simulink model "VELOCIDAD_COMP"  (R2015a)
settings: Solver=ode3  SolverMode=SingleTasking  StartTime=0.0  StopTime=inf  RelTol=1e-3
InitFcn:
  | % Periodo de muestreo control
  | % Periodo de muestreo control logico
  | tc=ts;
  | % Periodo de muestreo registro
  | tr=5e-3;
  | % Radio de la rueda (m)
  | R=86.1e-3/2;
  | % Distancia entre ruedas (m)
  | W=0.160;
  | % Constante de tiempo de filtrado
  | Tf_vel=200e-3; % Velocidad
values from neighbouring files (symbols this model uses):
  Cd = K*(1+1/(Ti*sd)+(Td*sd)/(1+Td*sd/N))    [ControlP.m]    (also in dead_2015.m = minreal(Fd/Pd/(1-Fd)); p4_3_diseño_directo.m = minreal(F/(Pd-F*Pd)))
  Crd = Cd    [ControlP.m]    (also in dead_2015.m; p4_3_diseño_directo.m)
  ts = 0.5    [ControlP.m]    (also in ControlPID_RF.m = 0.005; dead_2015.m = 0.055)
undefined symbols (not defined in the file or in its folder): Normalized
libraries: legonxtlib x10, simulink x6
settings Model: SimulationMode=external  CovSFcnEnable=off  ExtModeTrigDuration=2  Creator=mogimenez  LastModifiedBy=201809800
settings DataIOCC: SignalLoggingSaveFormat=ModelDataLogs
settings OptimizationCC: ExpressionDepthLimit=2147483647  OptimizeModelRefInitCode=on  LifeSpan=1
settings DebuggingCC: UnderspecifiedInitializationDetection=Classic  MergeDetectMultiDrivingBlocksExec=none  FcnCallInpInsideContextMsg=EnableAllAsWarning  StateNameClashWarn=warning
settings HardwareCC: ProdLargestAtomicInteger=Long  ProdLargestAtomicFloat=Float  ProdEndianess=LittleEndian  ProdHWDeviceType=ARM Compatible->ARM 7
settings RTWCC: SystemTargetFile=realtime.tlc  GenerateMakefile=off  TemplateMakefile=realtime.tmf  Description=Real-Time Toolbox  RTWVerbose=off
settings CodeAppCC: CustomSymbolStrType=$N$R$M  InternalIdentifier=Classic
settings ERTTargetCC: CombineOutputUpdateFcns=off  ExtMode=on  ExtModeTransport=1  ExtModeMexArgs=0 3 9600  InlinedParameterPlacement=Hierarchical  ERTSrcFileBannerTemplate=realtime_code_template.cgt  ERTHdrFileBannerTemplate=realtime_code_template.cgt  ERTDataSrcFileTemplate=realtime_code_template.cgt  ERTDataHdrFileTemplate=realtime_code_template.cgt  ERTCustomFileTemplate=realtime_file_process.tlc

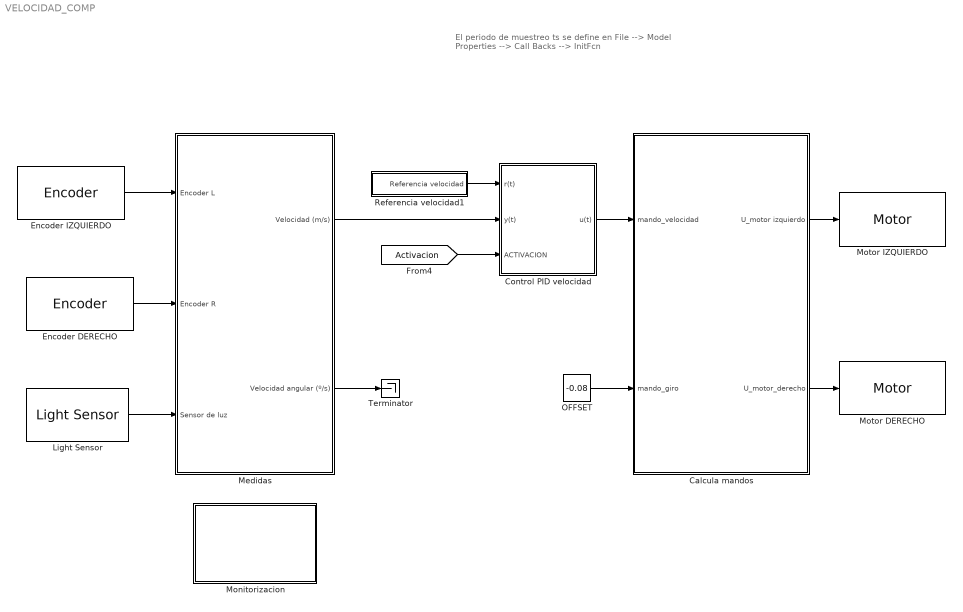
== system VELOCIDAD_COMP ==
  note: El periodo de muestreo ts se define en
      | File --> Model Properties --> Call Backs --> InitFcn
  Calcula mandos : Subsystem
  Control PID velocidad : Subsystem
  Encoder DERECHO : legonxtlib/Encoder  portNumber=C  opMode=No reset  sampleTime=tr  blockPlatform=LegoMindstormsNXT
  Encoder IZQUIERDO : legonxtlib/Encoder  portNumber=B  opMode=No reset  sampleTime=tr  blockPlatform=LegoMindstormsNXT
  Light Sensor : legonxtlib/Light Sensor  portNumber=4  outputMode=Normalized (0 -100)  lightOn=on  sampleTime=tc  blockPlatform=LegoMindstormsNXT
  Medidas : Subsystem
  Monitorizacion : Subsystem
  Motor DERECHO : legonxtlib/Motor  sportNumber=C  sstopAction=Brake  blockPlatform=LegoMindstormsNXT
  Motor IZQUIERDO : legonxtlib/Motor  sportNumber=B  sstopAction=Brake  blockPlatform=LegoMindstormsNXT
  OFFSET : Constant  Value=-0.08  SampleTime=ts
  Referencia velocidad1 : Subsystem  mask{Vmax=0.15, Vmin=0.1, T=2}
      mask prompts: Vmax "Valor maximo"; Vmin "Valor minimo"; T "Periodo (s)"
  Terminator : Terminator
  wires:
  Encoder DERECHO/1 -> Medidas/2(Encoder R)
  [Activacion] -> Control PID velocidad/3(ACTIVACION)
  Calcula mandos/1(U_motor izquierdo) -> Motor IZQUIERDO/1
  Calcula mandos/2(U_motor_derecho) -> Motor DERECHO/1
  Referencia velocidad1/1(Referencia velocidad) -> Control PID velocidad/1(r(t))
  Control PID velocidad/1(u(t)) -> Calcula mandos/1(mando_velocidad)
  Medidas/1(Velocidad (m/s)) -> Control PID velocidad/2(y(t))
  Encoder IZQUIERDO/1 -> Medidas/1(Encoder L)
  Light Sensor/1 -> Medidas/3(Sensor de luz)
  OFFSET/1 -> Calcula mandos/2(mando_giro)
  Medidas/2(Velocidad angular (º/s)) -> Terminator/1

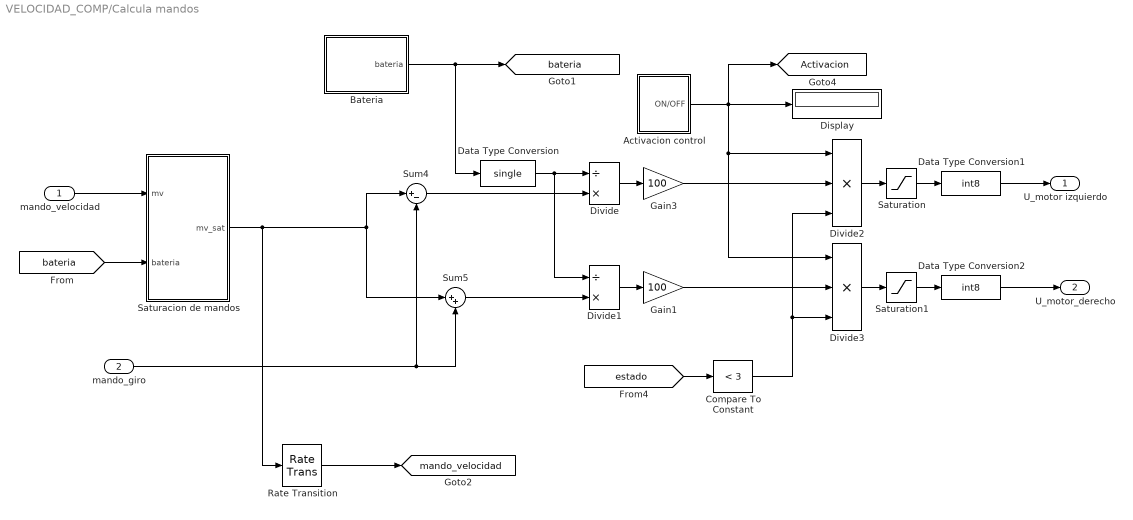
== system VELOCIDAD_COMP/Calcula mandos ==
  mando_velocidad : Inport
  mando_giro : Inport  Port=2
  Activacion control : Subsystem
  Bateria : Subsystem
  Compare To Constant : simulink/Logic and Bit Operations/Compare To Constant  relop=<  const=3  OutDataTypeStr=boolean
  Data Type Conversion : DataTypeConversion  OutDataTypeStr=single  SampleTime=ts
  Data Type Conversion1 : DataTypeConversion  OutDataTypeStr=int8
  Data Type Conversion2 : DataTypeConversion  OutDataTypeStr=int8
  Display : Display
  Divide : Product  Inputs=/*
  Divide1 : Product  Inputs=/*
  Divide2 : Product  Inputs=3  SampleTime=ts
  Divide3 : Product  Inputs=3  SampleTime=ts
  Gain1 : Gain  Gain=100
  Gain3 : Gain  Gain=100
  Rate Transition : RateTransition  OutPortSampleTime=tr
  Saturacion de mandos : Subsystem
  Saturation : Saturate  UpperLimit=100  LowerLimit=-100
  Saturation1 : Saturate  UpperLimit=100  LowerLimit=-100
  Sum4 : Sum  Inputs=|+-
  Sum5 : Sum  Inputs=|++
  U_motor izquierdo : Outport
  U_motor_derecho : Outport  Port=2
  tag scope: Activacion=global, bateria=global, mando_velocidad=global
  wires:
  Divide/1 -> Gain3/1
  Sum4/1 -> Divide/2
  Divide1/1 -> Gain1/1
  Sum5/1 -> Divide1/2
  Saturacion de mandos/1(mv_sat) -> Sum4/1, Sum5/1, Rate Transition/1
  mando_giro/1 -> Sum4/2, Sum5/2
  Bateria/1(bateria) -> Data Type Conversion/1, [bateria]
  Divide2/1 -> Saturation/1
  Divide3/1 -> Saturation1/1
  Activacion control/1(ON/OFF) -> Display/1, Divide2/1, Divide3/1, [Activacion]
  Data Type Conversion/1 -> Divide/1, Divide1/1
  Saturation/1 -> Data Type Conversion1/1
  Saturation1/1 -> Data Type Conversion2/1
  [bateria] -> Saturacion de mandos/2(bateria)
  Gain3/1 -> Divide2/2
  Gain1/1 -> Divide3/2
  mando_velocidad/1 -> Saturacion de mandos/1(mv)
  Data Type Conversion1/1 -> U_motor izquierdo/1
  Data Type Conversion2/1 -> U_motor_derecho/1
  Rate Transition/1 -> [mando_velocidad]
  [estado] -> Compare To Constant/1
  Compare To Constant/1 -> Divide2/3, Divide3/3

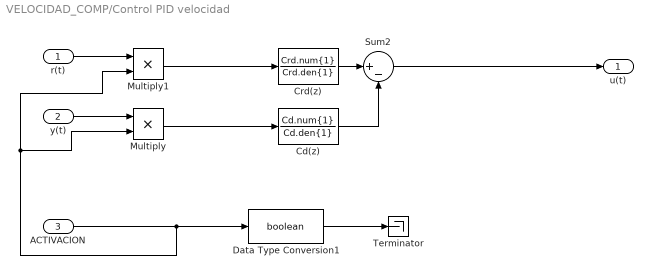
== system VELOCIDAD_COMP/Control PID velocidad ==
  r(t) : Inport  SampleTime=ts
  y(t) : Inport  Port=2  SampleTime=ts
  ACTIVACION : Inport  Port=3  SampleTime=ts
  Cd(z) : DiscreteTransferFcn  Numerator=Cd.num{1}  Denominator=Cd.den{1}  SampleTime=ts
  "Crd(z) " : DiscreteTransferFcn  Numerator=Crd.num{1}  Denominator=Crd.den{1}  SampleTime=ts
  Data Type Conversion1 : DataTypeConversion  OutDataTypeStr=boolean
  Multiply : Product  Inputs=**
  Multiply1 : Product  Inputs=**
  Sum2 : Sum  Inputs=|+-
  Terminator : Terminator
  u(t) : Outport
  wires:
  ACTIVACION/1 -> Multiply1/2, Multiply/2, Data Type Conversion1/1
  Data Type Conversion1/1 -> Terminator/1
  "Crd(z) "/1 -> Sum2/1
  Cd(z)/1 -> Sum2/2
  Sum2/1 -> u(t)/1
  y(t)/1 -> Multiply/1
  Multiply/1 -> Cd(z)/1
  r(t)/1 -> Multiply1/1
  Multiply1/1 -> "Crd(z) "/1

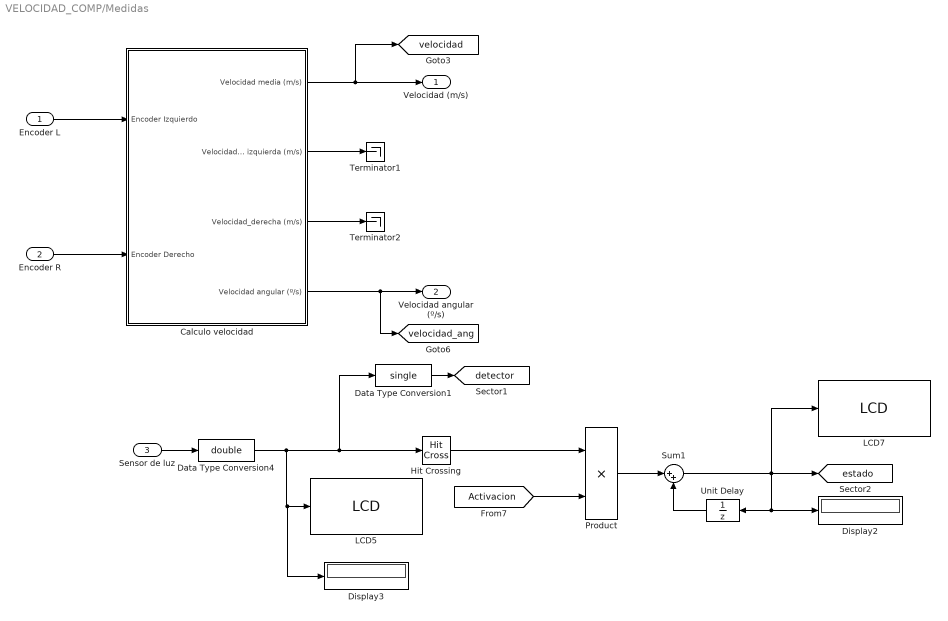
== system VELOCIDAD_COMP/Medidas ==
  Encoder L : Inport
  Encoder R : Inport  Port=2
  Sensor de luz : Inport  Port=3
  Calculo velocidad : Subsystem
  Data Type Conversion1 : DataTypeConversion  OutDataTypeStr=single  SampleTime=ts
  Data Type Conversion4 : DataTypeConversion  OutDataTypeStr=double  SampleTime=ts
  Display2 : Display
      settings: Decimation=50
  Display3 : Display
      settings: Decimation=50
  Hit Crossing : HitCross  HitCrossingOffset=44.5  HitCrossingDirection=falling
  LCD5 : legonxtlib/LCD  slcdStr=DETECT  slcdLine=2  slcdFormat=Decimal  blockPlatform=LegoMindstormsNXT
  LCD7 : legonxtlib/LCD  slcdStr=ESTADO  slcdLine=3  slcdFormat=Decimal  blockPlatform=LegoMindstormsNXT
  Product : Product  SampleTime=ts  RndMeth=Zero
  Sum1 : Sum  Inputs=|++
  Terminator1 : Terminator
  Terminator2 : Terminator
  Unit Delay : UnitDelay  InitialCondition=1  SampleTime=ts
  Velocidad (m/s) : Outport
  Velocidad angular (º/s) : Outport  Port=2
  tag scope: detector=global, estado=global, velocidad=global, velocidad_ang=global
  wires:
  Encoder R/1 -> Calculo velocidad/2(Encoder Derecho)
  Encoder L/1 -> Calculo velocidad/1(Encoder Izquierdo)
  Calculo velocidad/1(Velocidad media (m/s)) -> Velocidad (m/s)/1, [velocidad]
  Calculo velocidad/4(Velocidad angular (º/s)) -> Velocidad angular (º/s)/1, [velocidad_ang]
  Calculo velocidad/2(Velocidad izquierda (m/s)) -> Terminator1/1
  Calculo velocidad/3(Velocidad_derecha (m/s)) -> Terminator2/1
  Sensor de luz/1 -> Data Type Conversion4/1
  Sum1/1 -> LCD7/1, [estado], Unit Delay/1, Display2/1
  [Activacion] -> Product/2
  Product/1 -> Sum1/1
  Data Type Conversion4/1 -> Data Type Conversion1/1, Hit Crossing/1, Display3/1, LCD5/1
  Unit Delay/1 -> Sum1/2
  Hit Crossing/1 -> Product/1
  Data Type Conversion1/1 -> [detector]

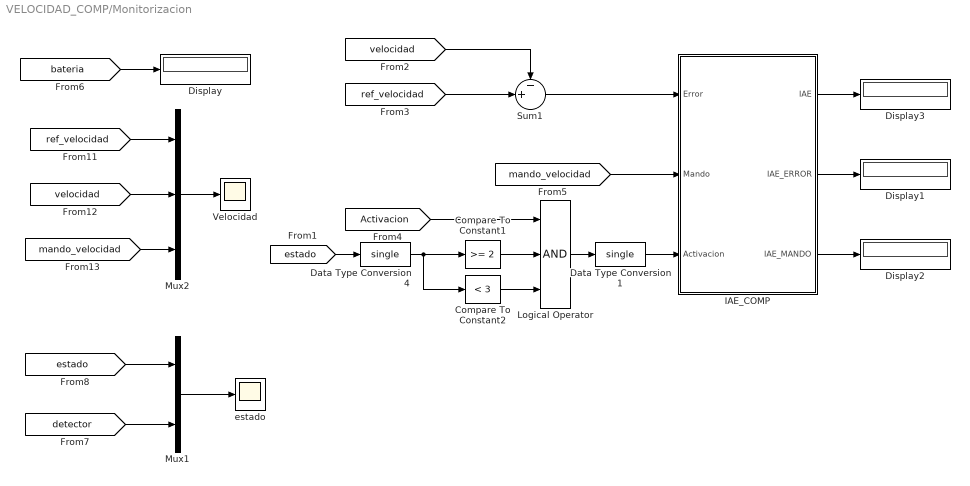
== system VELOCIDAD_COMP/Monitorizacion ==
  Compare To Constant1 : simulink/Logic and Bit Operations/Compare To Constant  relop=>=  const=2  OutDataTypeStr=uint8
  Compare To Constant2 : simulink/Logic and Bit Operations/Compare To Constant  relop=<  const=3  OutDataTypeStr=uint8
  Data Type Conversion1 : DataTypeConversion  OutDataTypeStr=single
  Data Type Conversion4 : DataTypeConversion  OutDataTypeStr=single
  Display{,1..3} (4 alike) : Display
      Display1 settings: Decimation=50
      Display2 settings: Decimation=50
      Display3 settings: Decimation=50
  IAE_COMP : Subsystem
      mask init:
      | SCALE = 300000;
      | FACTOR_MANDO = 2.5e-3;
  Logical Operator : Logic  Inputs=3  AllPortsSameDT=off  OutDataTypeStr=boolean
  Mux1 : Mux  Inputs=2
  Mux2 : Mux  Inputs=3
  Sum1 : Sum  Inputs=-+|  SampleTime=tr
  Velocidad : Scope
      settings: TimeRange=10  YMin=0  YMax=0.105  SaveName=Velocidad  SampleInput=on  SampleTime=tr
  estado : Scope
      settings: TimeRange=10  YMin=22.5  YMax=50  SaveName=estado  SampleInput=on  SampleTime=tr
  wires:
  [bateria] -> Display/1
  [ref_velocidad] -> Mux2/1
  [mando_velocidad] -> Mux2/3
  [velocidad] -> Mux2/2
  Mux2/1 -> Velocidad/1
  IAE_COMP/1(IAE) -> Display3/1
  Sum1/1 -> IAE_COMP/1(Error)
  Data Type Conversion4/1 -> Compare To Constant2/1, Compare To Constant1/1
  [estado] -> Data Type Conversion4/1
  Logical Operator/1 -> Data Type Conversion1/1
  [ref_velocidad] -> Sum1/2
  [velocidad] -> Sum1/1
  Compare To Constant1/1 -> Logical Operator/2
  Compare To Constant2/1 -> Logical Operator/3
  [estado] -> Mux1/1
  Mux1/1 -> estado/1
  [detector] -> Mux1/2
  Data Type Conversion1/1 -> IAE_COMP/3(Activacion)
  [Activacion] -> Logical Operator/1
  [mando_velocidad] -> IAE_COMP/2(Mando)
  IAE_COMP/2(IAE_ERROR) -> Display1/1
  IAE_COMP/3(IAE_MANDO) -> Display2/1

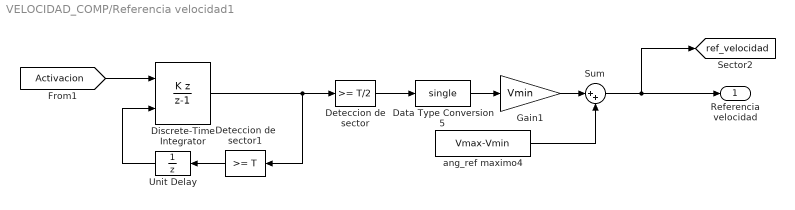
== system VELOCIDAD_COMP/Referencia velocidad1 ==
  Data Type Conversion5 : DataTypeConversion  OutDataTypeStr=single
  Deteccion de sector : simulink/Logic and Bit Operations/Compare To Constant  relop=>=  const=T/2  OutDataTypeStr=uint8
  Deteccion de sector1 : simulink/Logic and Bit Operations/Compare To Constant  relop=>=  const=T  OutDataTypeStr=uint8
  Discrete-Time Integrator : DiscreteIntegrator  IntegratorMethod=Accumulation: Backward Euler  gainval=tc  ExternalReset=rising  SampleTime=tc  OutDataTypeStr=single  UpperSaturationLimit=10  LowerSaturationLimit=0
  Gain1 : Gain  Gain=Vmin  ParamDataTypeStr=double  OutDataTypeStr=single
  Sum : Sum  Inputs=|++  SampleTime=ts
  Unit Delay : UnitDelay  SampleTime=tc
  ang_ref maximo4 : Constant  Value=Vmax-Vmin  OutDataTypeStr=single  SampleTime=tc
  Referencia velocidad : Outport  SampleTime=ts
  tag scope: ref_velocidad=global
  wires:
  ang_ref maximo4/1 -> Sum/2
  [Activacion] -> Discrete-Time Integrator/1
  Discrete-Time Integrator/1 -> Deteccion de sector1/1, Deteccion de sector/1
  Deteccion de sector/1 -> Data Type Conversion5/1
  Unit Delay/1 -> Discrete-Time Integrator/2
  Data Type Conversion5/1 -> Gain1/1
  Gain1/1 -> Sum/1
  Deteccion de sector1/1 -> Unit Delay/1
  Sum/1 -> [ref_velocidad], Referencia velocidad/1

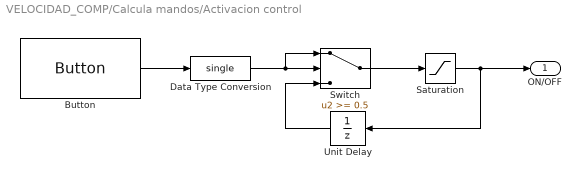
== system VELOCIDAD_COMP/Calcula mandos/Activacion control ==
  Button : legonxtlib/Button  buttonType=Middle orange  sampleTime=tc  blockPlatform=LegoMindstormsNXT
  Data Type Conversion : DataTypeConversion  OutDataTypeStr=single
  Saturation : Saturate  UpperLimit=1  LowerLimit=0
  Switch : Switch  Threshold=0.5
  Unit Delay : UnitDelay  SampleTime=tc
  ON/OFF : Outport
  wires:
  Button/1 -> Data Type Conversion/1
  Switch/1 -> Saturation/1
  Unit Delay/1 -> Switch/3
  Data Type Conversion/1 -> Switch/2, Switch/1
  Saturation/1 -> Unit Delay/1, ON/OFF/1

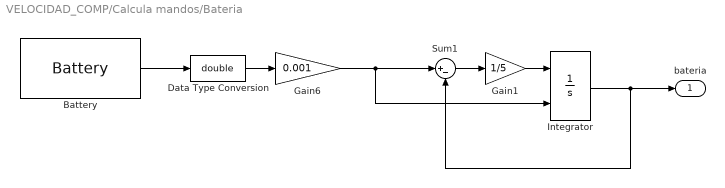
== system VELOCIDAD_COMP/Calcula mandos/Bateria ==
  Battery : legonxtlib/Battery  sampleTime=0.1  blockPlatform=LegoMindstormsNXT
  Data Type Conversion : DataTypeConversion  OutDataTypeStr=double
  Gain1 : Gain  Gain=1/5
  Gain6 : Gain  Gain=0.001
  Integrator : Integrator  InitialConditionSource=external
  Sum1 : Sum  Inputs=|+-
  bateria : Outport
  wires:
  Battery/1 -> Data Type Conversion/1
  Data Type Conversion/1 -> Gain6/1
  Sum1/1 -> Gain1/1
  Integrator/1 -> bateria/1, Sum1/2
  Gain6/1 -> Sum1/1, Integrator/2
  Gain1/1 -> Integrator/1

== system VELOCIDAD_COMP/Calcula mandos/Saturacion de mandos ==
  mv : Inport
  bateria : Inport  Port=2  SampleTime=ts
  Gain8 : Gain  Gain=-1
  Saturation Dynamic : simulink/Discontinuities/Saturation Dynamic  OutMin=[]  OutMax=[]  OutDataTypeStr=Inherit: Same as second input  OutDataType=fixdt(1, 16)  OutScaling=2^-10  DoSatur=off
  mv_sat : Outport
  wires:
  Gain8/1 -> Saturation Dynamic/3
  bateria/1 -> Gain8/1, Saturation Dynamic/1
  mv/1 -> Saturation Dynamic/2
  Saturation Dynamic/1 -> mv_sat/1

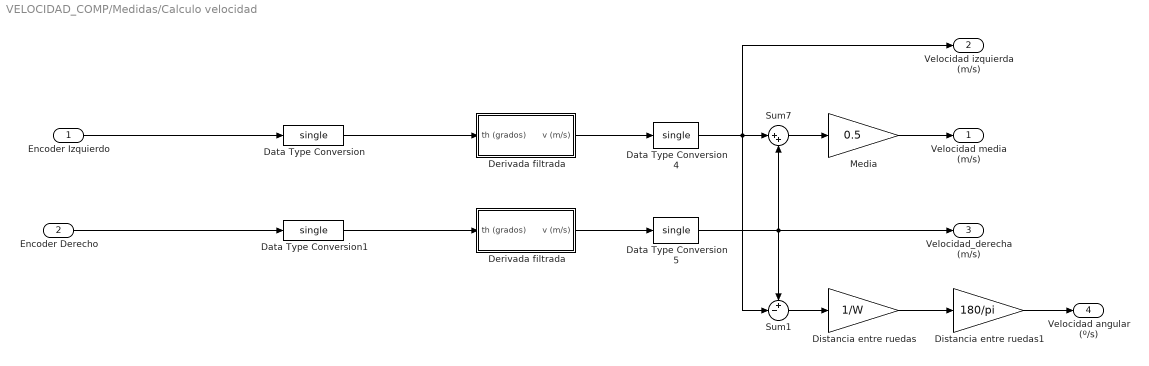
== system VELOCIDAD_COMP/Medidas/Calculo velocidad ==
  Encoder Izquierdo : Inport
  Encoder Derecho : Inport  Port=2
  Data Type Conversion{,1,4..5} (4 alike) : DataTypeConversion  OutDataTypeStr=single
  Derivada filtrada : Subsystem  mask{R=R, T=Tf_vel, ts=tr}
      mask prompts: R "Radio rueda (m)"; T "Constante de tiempo filtrado (s)"; ts "Periodo de muestreo"
      mask init:
      | alfa=exp(-ts/T);
  "Derivada filtrada " : Subsystem  mask{R=R, T=Tf_vel, ts=tr}
      mask prompts: R "Radio rueda (m)"; T "Constante de tiempo filtrado (s)"; ts "Periodo de muestreo"
      mask init:
      | alfa=exp(-ts/T);
  Distancia entre ruedas : Gain  Gain=1/W
  Distancia entre ruedas1 : Gain  Gain=180/pi
  Media : Gain  Gain=0.5
  Sum1 : Sum  Inputs=+-|
  Sum7 : Sum  Inputs=|++
  Velocidad media (m/s) : Outport
  Velocidad izquierda (m/s) : Outport  Port=2
  Velocidad_derecha (m/s) : Outport  Port=3
  Velocidad angular (º/s) : Outport  Port=4
  wires:
  Data Type Conversion1/1 -> Derivada filtrada/1(th (grados))
  Derivada filtrada/1(v (m/s)) -> Data Type Conversion5/1
  "Derivada filtrada "/1(v (m/s)) -> Data Type Conversion4/1
  Data Type Conversion4/1 -> Sum1/2, Velocidad izquierda (m/s)/1, Sum7/1
  Data Type Conversion5/1 -> Sum1/1, Velocidad_derecha (m/s)/1, Sum7/2
  Sum7/1 -> Media/1
  Media/1 -> Velocidad media (m/s)/1
  Data Type Conversion/1 -> "Derivada filtrada "/1(th (grados))
  Sum1/1 -> Distancia entre ruedas/1
  Distancia entre ruedas/1 -> Distancia entre ruedas1/1
  Distancia entre ruedas1/1 -> Velocidad angular (º/s)/1
  Encoder Izquierdo/1 -> Data Type Conversion/1
  Encoder Derecho/1 -> Data Type Conversion1/1

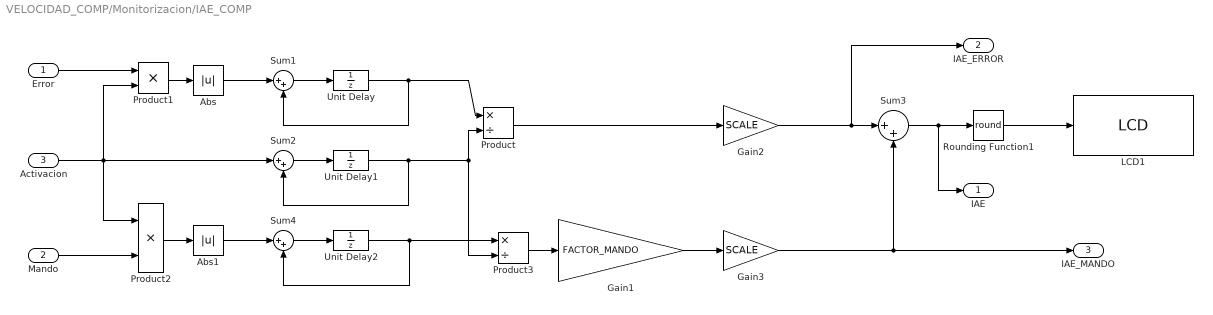
== system VELOCIDAD_COMP/Monitorizacion/IAE_COMP ==
  Error : Inport
  Mando : Inport  Port=2
  Activacion : Inport  Port=3
  Abs : Abs
  Abs1 : Abs
  Gain1 : Gain  Gain=FACTOR_MANDO
  Gain2 : Gain  Gain=SCALE
  Gain3 : Gain  Gain=SCALE
  LCD1 : legonxtlib/LCD  slcdStr=IAE  slcdLine=1  slcdFormat=Decimal  blockPlatform=LegoMindstormsNXT
  Product : Product  Inputs=*/  RndMeth=Zero
  Product1 : Product  RndMeth=Zero
  Product2 : Product  RndMeth=Zero
  Product3 : Product  Inputs=*/  RndMeth=Zero
  Rounding Function1 : Rounding  Operator=round
  Sum1 : Sum  Inputs=|++
  Sum2 : Sum  Inputs=|++
  Sum3 : Sum  Inputs=|++  SampleTime=tr
  Sum4 : Sum  Inputs=|++
  Unit Delay : UnitDelay  SampleTime=-1
  Unit Delay1 : UnitDelay  InitialCondition=1  SampleTime=-1
  Unit Delay2 : UnitDelay  SampleTime=-1
  IAE : Outport
  IAE_ERROR : Outport  Port=2
  IAE_MANDO : Outport  Port=3
  wires:
  Error/1 -> Product1/1
  Product1/1 -> Abs/1
  Activacion/1 -> Product2/1, Product1/2, Sum2/1
  Unit Delay1/1 -> Product3/2, Product/2, Sum2/2
  Sum2/1 -> Unit Delay1/1
  Unit Delay/1 -> Product/1, Sum1/2
  Sum1/1 -> Unit Delay/1
  Abs/1 -> Sum1/1
  Sum3/1 -> Rounding Function1/1, IAE/1
  Rounding Function1/1 -> LCD1/1
  Product/1 -> Gain2/1
  Gain1/1 -> Gain3/1
  Gain2/1 -> IAE_ERROR/1, Sum3/1
  Gain3/1 -> Sum3/2, IAE_MANDO/1
  Product2/1 -> Abs1/1
  Mando/1 -> Product2/2
  Unit Delay2/1 -> Product3/1, Sum4/2
  Sum4/1 -> Unit Delay2/1
  Abs1/1 -> Sum4/1
  Product3/1 -> Gain1/1

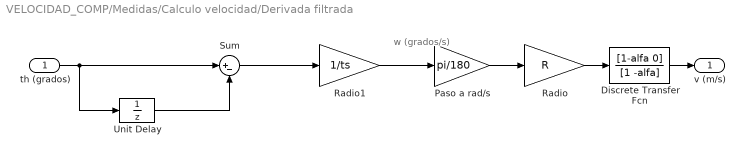
== system VELOCIDAD_COMP/Medidas/Calculo velocidad/Derivada filtrada ==
  note: w (grados/s)
  th (grados) : Inport  SampleTime=ts
  Discrete Transfer Fcn : DiscreteTransferFcn  Numerator=[1-alfa 0]  Denominator=[1 -alfa]
  Paso a rad/s : Gain  Gain=pi/180
  Radio : Gain  Gain=R
  Radio1 : Gain  Gain=1/ts
  Sum : Sum  Inputs=|+-
  Unit Delay : UnitDelay  SampleTime=-1
  v (m/s) : Outport
  wires:
  th (grados)/1 -> Unit Delay/1, Sum/1
  Unit Delay/1 -> Sum/2
  Sum/1 -> Radio1/1
  Radio1/1 -> Paso a rad/s/1
  Paso a rad/s/1 -> Radio/1
  Radio/1 -> Discrete Transfer Fcn/1
  Discrete Transfer Fcn/1 -> v (m/s)/1

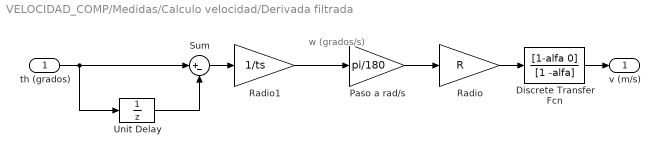
== system VELOCIDAD_COMP/Medidas/Calculo velocidad/Derivada filtrada  ==
  note: w (grados/s)
  th (grados) : Inport  SampleTime=ts
  Discrete Transfer Fcn : DiscreteTransferFcn  Numerator=[1-alfa 0]  Denominator=[1 -alfa]
  Paso a rad/s : Gain  Gain=pi/180
  Radio : Gain  Gain=R
  Radio1 : Gain  Gain=1/ts
  Sum : Sum  Inputs=|+-
  Unit Delay : UnitDelay  SampleTime=-1
  v (m/s) : Outport
  wires:
  Discrete Transfer Fcn/1 -> v (m/s)/1
  Radio/1 -> Discrete Transfer Fcn/1
  Paso a rad/s/1 -> Radio/1
  Radio1/1 -> Paso a rad/s/1
  Sum/1 -> Radio1/1
  Unit Delay/1 -> Sum/2
  th (grados)/1 -> Sum/1, Unit Delay/1
